simulink model "LabB_ObserverAndControllerOverRobot"  (R2023a)
settings: Solver=FixedStepDiscrete  StartTime=0.0  StopTime=inf  FixedStep=fSamplingPeriod  RelTol=1e-3  EnableMultiTasking=on
values from neighbouring files (symbols this model uses):
  Ad = [1 0 0 0 0.00216937580494 0.169257508882 0.0123862127288 3.63566071015 -3.56150302531e-05 -0.00954899425386 1.00059754622 0.218485145883 ... (16 elements, 4x4)]    [4_9.mat]    (also in IMPROVED_LQR_NUMRICAL.mat; LabB_ControllerOverSimulator_Discrete_Parameters.m = discreteStateSpace.A; LabB_ObserverAndControllerOverRobot_Parameters.m = [; LabB_ObserverAndControllerOverSimulator_Discrete_Parameters.m = discreteStateSpace.A)
  Bd = [0.000133880874091 0.0392918745799 -0.000585834385821 -0.17195692548]    [4_9.mat]    (also in IMPROVED_LQR_NUMRICAL.mat; LabB_ControllerOverSimulator_Discrete_Parameters.m = discreteStateSpace.B; LabB_ObserverAndControllerOverRobot_Parameters.m = [; LabB_ObserverAndControllerOverSimulator_Discrete_Parameters.m = discreteStateSpace.B)
  Cd = [1  0  0  0; 0  0  1  0]    [4_9.mat]    (also in IMPROVED_LQR_NUMRICAL.mat; LabB_ControllerOverSimulator_Discrete_Parameters.m = discreteStateSpace.C; LabB_ObserverAndControllerOverRobot_Parameters.m = [; LabB_ObserverAndControllerOverSimulator_Discrete_Parameters.m = discreteStateSpace.C)
  fGyroBias = -36.0405046481    [Copy_of_GyroBias.mat]    (also in GyroBias.mat; IMPROVED_LQR_NUMRICAL.mat = -55.293398533; PID_10_25.mat = -23.8864197531; PID_10_25_PROCESSED.mat = -23.8864197531)
  fGyroConversionFactor = 0.00762939453125    [IMPROVED_LQR_NUMRICAL.mat]    (also in LabB_ObserverAndControllerOverRobot_Parameters.m = -0.00763358778626; PID_10_25.mat = -0.00763358778626; PID_10_25_PROCESSED.mat = -0.00763358778626)
  fSamplingPeriod = 0.005    [4_10_numerical_derivative.mat]    (also in 4_9.mat; IMPROVED_LQR_NUMRICAL.mat; LabB_ControllerOverSimulator_Discrete_Parameters.m; LabB_ObserverAndControllerOverRobot_Parameters.m = 0.05)
  fWheelRadius = 0.0216    [IMPROVED_LQR_NUMRICAL.mat]    (also in LabB_ObserverAndControllerOverRobot_Parameters.m; PID_10_25.mat; PID_10_25_PROCESSED.mat)
  iNumberOfEncoderSteps = 720    [IMPROVED_LQR_NUMRICAL.mat]    (also in LabB_ObserverAndControllerOverRobot_Parameters.m; PID_10_25.mat; PID_10_25_PROCESSED.mat)
  Kd = -0.0902330229907    [4_8.mat]    (also in 4_8_LQR.mat; 4_9.mat = [-21.5910873349 -42.5517839322 -61.6884020442 -10.1567027547; IMPROVED_LQR_NUMRICAL.mat = [-21.5910873363 -42.5517839322 -61.6884020444 -10.1567027547; LabB_ControllerOverSimulator_Discrete_Parameters.m = acker(Ad,Bd,discretePoles))
  Ld = [0.113484873259  0.00523048580375; -1.36818722201  4.37324641743; 0.0236786814247  0.320119081479; 6.39094177477  -15.2655028264]    [4_9.mat]    (also in IMPROVED_LQR_NUMRICAL.mat = [0.14317878514  0.00902187336613; -0.912440934111  2.0839431; LabB_ObserverAndControllerOverRobot_Parameters.m = [; LabB_ObserverAndControllerOverSimulator_Discrete_Parameters.m = (place(Ad',Cd',desiredPoles))'; LabB_ObserverOverSimulator_Discrete_Parameters.m = (place(Ad',Cd',desiredPoles))')
  Md1 = [0.818659998491  0.0205458327288  0.00496425143631; 0.0212966370717  0.986017031865  0.0397631461808; -0.0224685177823  -0.180533078124  0.819806639231]    [4_9.mat]    (also in IMPROVED_LQR_NUMRICAL.mat = [0.852155353499  -0.0520013200777  0.00297877258471; -0.0532; LabB_ObserverAndControllerOverRobot_Parameters.m = [; LabB_ObserverAndControllerOverSimulator_Discrete_Parameters.m = Axx-Lacc*Ayx-Lnacc*Cx; LabB_ObserverOverSimulator_Discrete_Parameters.m = Axx-Lacc*Ayx-Lnacc*Cx)
  Md2 = [-8.22715382193e-05 0.0896973776791 -0.407469536485]    [4_9.mat]    (also in IMPROVED_LQR_NUMRICAL.mat = [-0.00455944705037 0.0553880900201 -0.371633068277]; LabB_ObserverAndControllerOverRobot_Parameters.m = [; LabB_ObserverAndControllerOverSimulator_Discrete_Parameters.m = Bx-Lacc*By; LabB_ObserverOverSimulator_Discrete_Parameters.m = Bx-Lacc*By)
  Md3 = [3.76127546986 376.495174844 -1759.12065562]    [4_9.mat]    (also in IMPROVED_LQR_NUMRICAL.mat = [-29.6802115428 120.227893263 -1491.44636344]; LabB_ObserverAndControllerOverRobot_Parameters.m = 1.0e+03 * [; LabB_ObserverAndControllerOverSimulator_Discrete_Parameters.m = Axy-Lacc*Ayy-Lnacc*Cy; LabB_ObserverOverSimulator_Discrete_Parameters.m = Axy-Lacc*Ayy-Lnacc*Cy)
  Md4 = [0.181803589786 -0.0442545183678 0.303604799034]    [4_9.mat]    (also in IMPROVED_LQR_NUMRICAL.mat = [0.14949925435 0.0394504885475 0.221851502925]; LabB_ObserverAndControllerOverRobot_Parameters.m = [; LabB_ObserverAndControllerOverSimulator_Discrete_Parameters.m = Lnacc; LabB_ObserverOverSimulator_Discrete_Parameters.m = Lnacc)
  Md5 = [-3.76127546986 -376.495174844 1759.12065562]    [4_9.mat]    (also in IMPROVED_LQR_NUMRICAL.mat = [29.6802115428 -120.227893263 1491.44636344]; LabB_ObserverAndControllerOverRobot_Parameters.m = 1.0e+03 * [; LabB_ObserverAndControllerOverSimulator_Discrete_Parameters.m = Lacc; LabB_ObserverOverSimulator_Discrete_Parameters.m = Lacc)
  Md6 = [1 0 0 0]    [4_9.mat]    (also in IMPROVED_LQR_NUMRICAL.mat; LabB_ObserverAndControllerOverRobot_Parameters.m = [; LabB_ObserverAndControllerOverSimulator_Discrete_Parameters.m = T(:,1); LabB_ObserverOverSimulator_Discrete_Parameters.m = T(:,1))
  Md7 = [0  0  0; 0  1  0; 1  0  0; 0  0  1]    [4_9.mat]    (also in IMPROVED_LQR_NUMRICAL.mat; LabB_ObserverAndControllerOverRobot_Parameters.m = [; LabB_ObserverAndControllerOverSimulator_Discrete_Parameters.m = T(:,2:4); LabB_ObserverOverSimulator_Discrete_Parameters.m = T(:,2:4))
undefined symbols (not defined in the file or in its folder): DiscIntNeverNeededParam
libraries: simulink x16, cstblocks x2, MinSegLibrary_M2V3 x2, arduinolib x1
settings Model: FPTRunName=FPA_Reference  SimulationMode=external  ExtModeTrigDuration=2  Creator=Alec  LastModifiedBy=Jasminis
settings SolverCC: AlgebraicLoopSolver=TrustRegion
settings DataIOCC: SaveFormat=Array  SaveOutput=off  SignalLogging=off  DSMLogging=off  SaveTime=off  ReturnWorkspaceOutputs=off
settings OptimizationCC: PassReuseOutputArgsAs=Individual arguments  ExpressionDepthLimit=2147483647  MaxStackSize=64  EfficientTunableParamExpr=on
settings DebuggingCC: UnderspecifiedInitializationDetection=Classic  MergeDetectMultiDrivingBlocksExec=none  ParameterTunabilityLossMsg=error  UnconnectedInputMsg=warning  UnconnectedOutputMsg=warning  UnconnectedLineMsg=warning  StateNameClashWarn=warning  SFUnexpectedBacktrackingDiag=warning  SFNoUnconditionalDefaultTransitionDiag=warning  SFExecutionAtInitializationDiag=none  ArithmeticOperatorsInVariantConditions=warning
settings HardwareCC: ProdBitPerInt=16  ProdBitPerPointer=16  ProdBitPerSizeT=16  ProdBitPerPtrDiffT=16  ProdLargestAtomicFloat=None  ProdWordSize=8  ProdHWDeviceType=Atmel->AVR
settings ModelReferenceCC: EnableRefExpFcnMdlSchedulingChecks=on  PropagateSignalLabelsOutOfModel=off
settings SFSimCC: SimUseLocalCustomCode=off  MATLABDynamicMemAlloc=off  CustomCodeUndefinedFunction=UseInterfaceOnly
settings RTWCC: Description=Embedded Coder  SystemTargetFile=ert.tlc  HardwareBoard=Arduino Mega 2560  TemplateMakefile=ert_default_tmf  GenerateReport=on  RTWVerbose=off  RTWUseLocalCustomCode=off  Toolchain=Arduino AVR  BuildConfiguration=Faster Runs  IncludeHyperlinkInReport=on  LaunchReport=on  GenerateTraceInfo=on  GenerateTraceReport=on  GenerateTraceReportSl=on  GenerateTraceReportSf=on  GenerateTraceReportEml=on
settings CodeAppCC: ForceParamTrailComments=on  IgnoreCustomStorageClasses=off  OperatorAnnotations=on  SimulinkDataObjDesc=on  SFDataObjDesc=on  MATLABFcnDesc=on  CustomSymbolStrType=$N$R$M  InsertBlockDesc=on  StateflowObjectComments=on  MATLABSourceComments=on  InternalIdentifier=Classic
settings ERTTargetCC: SupportContinuousTime=on  SupportVariableSizeSignals=on
settings ConfigComp: CovMetricSettings=dw  CovSaveCumulativeToWorkspaceVar=on  CovSaveSingleToWorkspaceVar=on  CovExternalEMLEnable=off

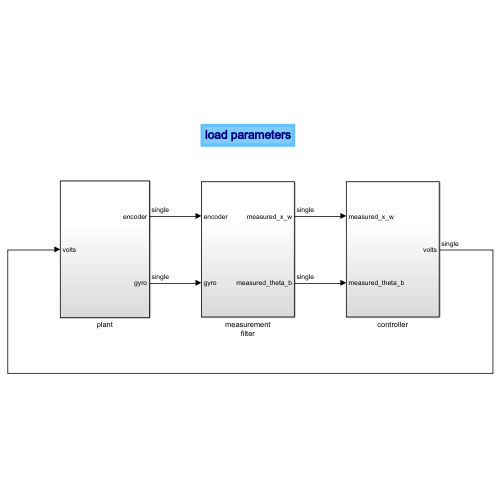
[thumbnail: Simulink's stored preview of the top-level diagram]
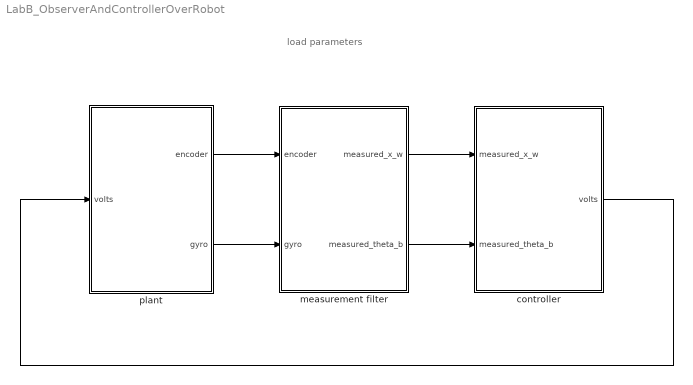
== system LabB_ObserverAndControllerOverRobot ==
  note: load parameters
  controller : Subsystem
  measurement filter : Subsystem
  plant : Subsystem
  wires:
  plant/2(gyro) -> measurement filter/2(gyro)
  measurement filter/2(measured_theta_b) -> controller/2("measured_theta_b ")
  measurement filter/1(measured_x_w) -> controller/1(measured_x_w)
  plant/1(encoder) -> measurement filter/1(encoder)
  controller/1(volts) -> plant/1(volts)

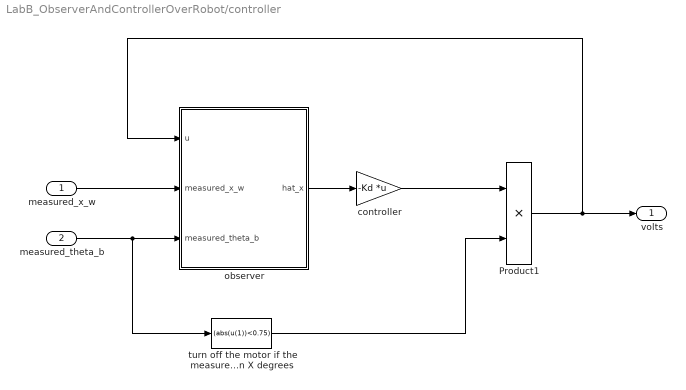
== system LabB_ObserverAndControllerOverRobot/controller ==
  measured_x_w : Inport
  "measured_theta_b " : Inport  Port=2
  Product1 : Product  RndMeth=Zero
  controller : Gain  Gain=-Kd  Multiplication=Matrix(K*u)
  observer : Subsystem
  turn off the motor if the measured angle is greater than X degrees : Fcn  Expr=(abs(u(1))<0.75)
  volts : Outport
  wires:
  observer/1(hat_x) -> controller/1
  turn off the motor if the measured angle is greater than X degrees/1 -> Product1/2
  "measured_theta_b "/1 -> observer/3(measured_theta_b), turn off the motor if the measured angle is greater than X degrees/1
  controller/1 -> Product1/1
  measured_x_w/1 -> observer/2(measured_x_w)
  Product1/1 -> observer/1(u), volts/1

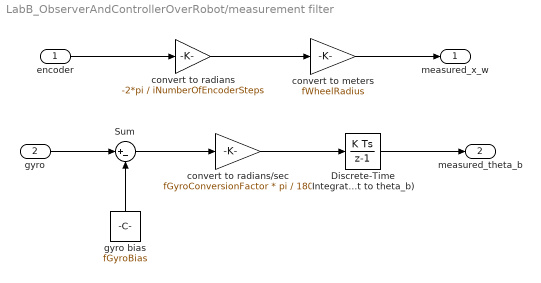
== system LabB_ObserverAndControllerOverRobot/measurement filter ==
  encoder : Inport
  gyro : Inport  Port=2
  Discrete-Time Integrator (convert from theta_b_dot to theta_b) : DiscreteIntegrator  SampleTime=fSamplingPeriod  OutDataTypeStr=Inherit: Inherit via back propagation  ICPrevOutput=DiscIntNeverNeededParam  ICPrevScaledInput=DiscIntNeverNeededParam
  Sum : Sum  Inputs=|+-
  convert to radians/sec : Gain  Gain=fGyroConversionFactor * pi / 180  OutDataTypeStr=Inherit: Same as input
  convert to radians : Gain  Gain=-2*pi / iNumberOfEncoderSteps  OutDataTypeStr=Inherit: Same as input
  convert to meters : Gain  Gain=fWheelRadius  OutDataTypeStr=Inherit: Same as input
  gyro bias : Constant  Value=fGyroBias  OutDataTypeStr=single
  measured_x_w : Outport
  measured_theta_b : Outport  Port=2
  wires:
  convert to radians/sec/1 -> Discrete-Time Integrator (convert from theta_b_dot to theta_b)/1
  gyro/1 -> Sum/1
  Sum/1 -> convert to radians/sec/1
  convert to radians/1 -> convert to meters/1
  encoder/1 -> convert to radians/1
  Discrete-Time Integrator (convert from theta_b_dot to theta_b)/1 -> measured_theta_b/1
  gyro bias/1 -> Sum/2
  convert to meters/1 -> measured_x_w/1

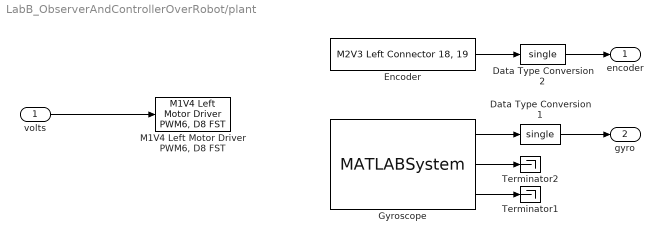
== system LabB_ObserverAndControllerOverRobot/plant ==
  volts : Inport
  Data Type Conversion1 : DataTypeConversion  OutDataTypeStr=single  SaturateOnIntegerOverflow=off  RndMeth=Floor
  Data Type Conversion2 : DataTypeConversion  OutDataTypeStr=single  SaturateOnIntegerOverflow=off  RndMeth=Floor
  Encoder : MinSegLibrary_M2V3/M2V3 Left Connector 18, 19  Encoder=1  PinA=19  PinB=18
      settings: SourceProductName=Rensselaer Arduino Support Package
  Gyroscope : MATLABSystem  System=soMPU6050Gyro  DLPFmode=0
      mask Type: soMPU6050Gyro
      mask Display:
      | disp('soMPU6050Gyro');
      | port_label('output',1,'xvel');
      | port_label('output',2,'yvel');
      | port_label('output',3,'zvel');
  "M1V4 Left Motor Driver PWM6, D8 FST" : MinSegLibrary_M2V3/M1V4 Left Motor Driver PWM6, D8 FST  Vsupply=9
      settings: SourceProductName=Rensselaer Arduino Support Package
  Terminator1 : Terminator
  Terminator2 : Terminator
  encoder : Outport
  gyro : Outport  Port=2
  wires:
  Gyroscope/1 -> Data Type Conversion1/1
  Data Type Conversion1/1 -> gyro/1
  Encoder/1 -> Data Type Conversion2/1
  Data Type Conversion2/1 -> encoder/1
  Gyroscope/3 -> Terminator1/1
  Gyroscope/2 -> Terminator2/1
  volts/1 -> "M1V4 Left Motor Driver PWM6, D8 FST"/1

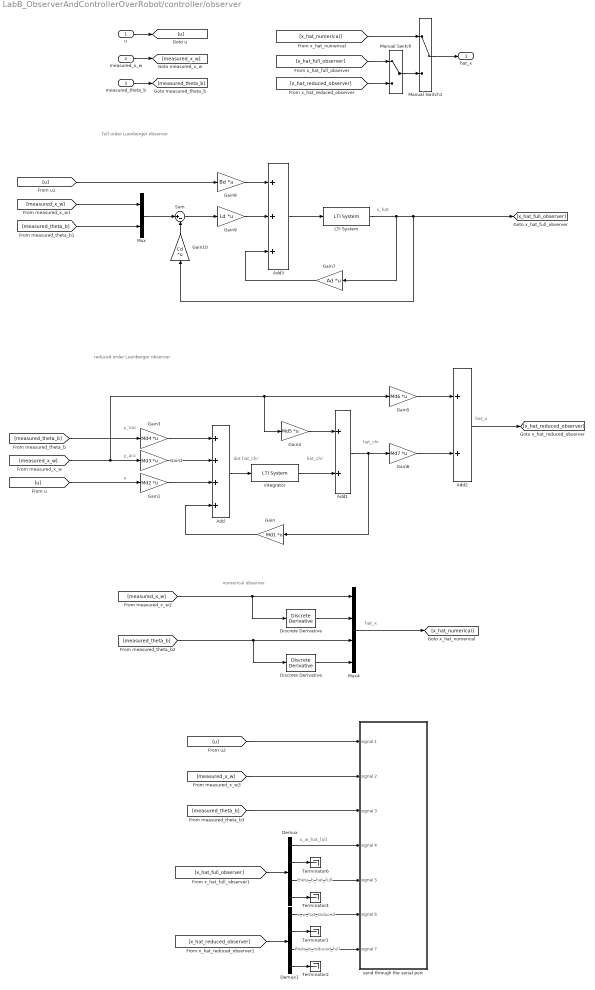
== system LabB_ObserverAndControllerOverRobot/controller/observer ==
  note: x_w_hat_full
  note: full order Luenberger observer
  note: reduced order Luenberger observer
  note: numerical observer
  note: hat_x
  note: hat_chi
  note: u
  note: dot hat_chi'
  note: hat_chi'
  note: y_acc
  note: y_nac
  note: x_hat
  note: hat_x
  note: x_w_hat_reduced
  note: theta_b_hat_full
  note: theta_b_reduced_full
  u : Inport
  measured_x_w : Inport  Port=2
  measured_theta_b : Inport  Port=3
  Add : Sum  Inputs=++++
  Add1 : Sum
  Add2 : Sum
  Add3 : Sum  Inputs=+++
  Demux : Demux
  Demux1 : Demux
  Discrete Derivative : simulink/Discrete/Discrete Derivative  gainval=1.0  ICPrevScaledInput=0.0  OutMin=[]  OutMax=[]  OutDataType=fixdt(1, 16)  OutScaling=2^-10  DoSatur=off
  "Discrete Derivative " : simulink/Discrete/Discrete Derivative  gainval=1.0  ICPrevScaledInput=0.0  OutMin=[]  OutMax=[]  OutDataType=fixdt(1, 16)  OutScaling=2^-10  DoSatur=off
  Gain : Gain  Gain=Md1  Multiplication=Matrix(K*u)
  Gain1 : Gain  Gain=Md2  Multiplication=Matrix(K*u)
  Gain10 : Gain  Gain=Cd  Multiplication=Matrix(K*u)
  Gain2 : Gain  Gain=Md3  Multiplication=Matrix(K*u)
  Gain3 : Gain  Gain=Md4  Multiplication=Matrix(K*u)
  Gain4 : Gain  Gain=Md5  Multiplication=Matrix(K*u)
  Gain5 : Gain  Gain=Md6  Multiplication=Matrix(K*u)
  Gain6 : Gain  Gain=Md7  Multiplication=Matrix(K*u)
  Gain7 : Gain  Gain=Ad  Multiplication=Matrix(K*u)
  Gain8 : Gain  Gain=Bd  Multiplication=Matrix(K*u)
  Gain9 : Gain  Gain=Ld  Multiplication=Matrix(K*u)
  LTI System : cstblocks/LTI System  sys=tf(1,[1 0],fSamplingPeriod)*eye(size(Ad))  IC=[]
  Manual Switch : ManualSwitch
  Manual Switch1 : ManualSwitch
  Mux : Mux  Inputs=2
  Mux4 : Mux
  Sum : Sum  Inputs=|+-
  Terminator{1..2,4,6} (4 alike) : Terminator
  integrator : cstblocks/LTI System  sys=tf(1,[1 0],fSamplingPeriod)*eye(3)  IC=[]
  send through the serial port : Subsystem
  hat_x : Outport
  wires:
  Gain3/1 -> Add/1
  Gain2/1 -> Add/2
  Add/1 -> integrator/1
  Gain4/1 -> Add1/1
  Gain1/1 -> Add/3
  Gain/1 -> Add/4
  integrator/1 -> Add1/2
  Add1/1 -> Gain/1, Gain6/1
  Gain5/1 -> Add2/1
  Gain6/1 -> Add2/2
  Discrete Derivative/1 -> Mux4/2
  "Discrete Derivative "/1 -> Mux4/4
  [measured_x_w] -> Gain4/1, Gain5/1, Gain2/1
  [measured_theta_b] -> Gain3/1
  Gain9/1 -> Add3/2
  Sum/1 -> Gain9/1
  [u] -> Gain1/1
  Gain8/1 -> Add3/1
  Gain10/1 -> Sum/2
  Mux/1 -> Sum/1
  Gain7/1 -> Add3/3
  LTI System/1 -> [x_hat_full_observer], Gain10/1, Gain7/1
  Add3/1 -> LTI System/1
  u/1 -> [u]
  measured_x_w/1 -> [measured_x_w]
  measured_theta_b/1 -> [measured_theta_b]
  [u] -> Gain8/1
  [measured_x_w] -> Mux/1
  [measured_theta_b] -> Mux/2
  [measured_x_w] -> Discrete Derivative/1, Mux4/1
  [measured_theta_b] -> "Discrete Derivative "/1, Mux4/3
  [u] -> send through the serial port/1(signal 1)
  [measured_x_w] -> send through the serial port/2(signal 2)
  [measured_theta_b] -> send through the serial port/3(signal 3)
  Mux4/1 -> [x_hat_numerical]
  [x_hat_full_observer] -> Manual Switch/1
  Manual Switch/1 -> Manual Switch1/2
  Manual Switch1/1 -> hat_x/1
  Add2/1 -> [x_hat_reduced_observer]
  [x_hat_reduced_observer] -> Manual Switch/2
  [x_hat_numerical] -> Manual Switch1/1
  [x_hat_full_observer] -> Demux/1
  Demux/1 -> send through the serial port/4(signal 4)
  Demux/3 -> send through the serial port/5(signal 5)
  Demux1/3 -> send through the serial port/7(signal 7)
  Demux1/1 -> send through the serial port/6(signal 6)
  [x_hat_reduced_observer] -> Demux1/1
  Demux/2 -> Terminator6/1
  Demux/4 -> Terminator4/1
  Demux1/2 -> Terminator1/1
  Demux1/4 -> Terminator2/1

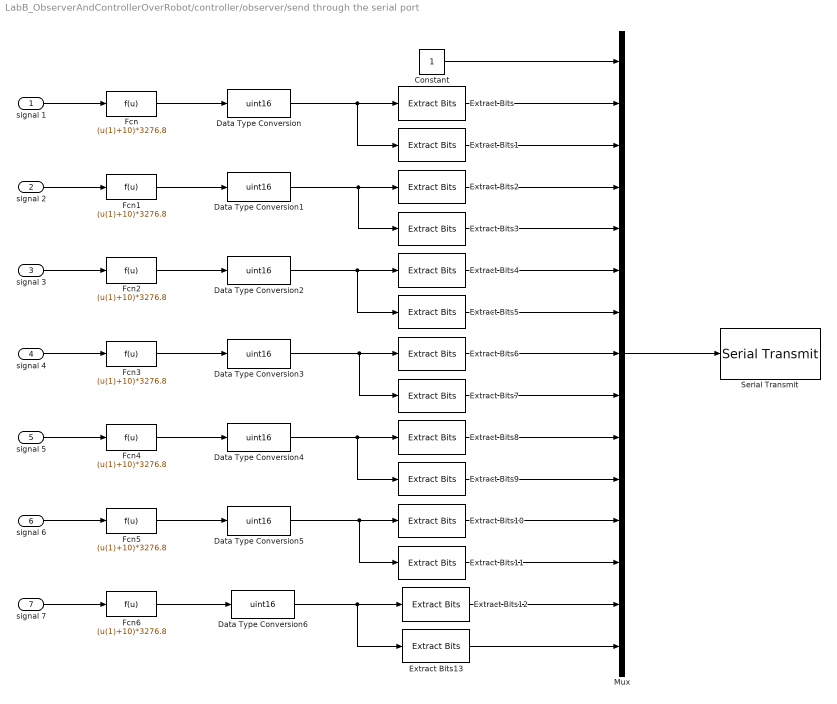
== system LabB_ObserverAndControllerOverRobot/controller/observer/send through the serial port ==
  signal 1 : Inport
  signal 2 : Inport  Port=2
  signal 3 : Inport  Port=3
  signal 4 : Inport  Port=4
  signal 5 : Inport  Port=5
  signal 6 : Inport  Port=6
  signal 7 : Inport  Port=7
  Constant : Constant  OutDataTypeStr=uint8
  Data Type Conversion{,1..6} (7 alike) : DataTypeConversion  OutDataTypeStr=uint16  SaturateOnIntegerOverflow=off  RndMeth=Floor
  Extract Bits{,2,4,6,8,10,12} (7 alike) : simulink/Logic and Bit Operations/Extract Bits  bitsToExtract=Upper half  numBits=8  bitIdxRange=[0 7]  outScalingMode=Treat bit field as an integer
  Extract Bits{1,3,5,7,9,11,13} (7 alike) : simulink/Logic and Bit Operations/Extract Bits  bitsToExtract=Lower half  numBits=8  bitIdxRange=[0 7]  outScalingMode=Treat bit field as an integer
  Fcn{,1..6} (7 alike) : Fcn  Expr=(u(1)+10)*3276.8
  Mux : Mux  Inputs=15
  Serial Transmit : arduinolib/Serial Transmit  portNumber=0  sendmode=write  sendformat=Decimal  floatprecision=2  blockPlatform=arduino
  wires:
  Data Type Conversion/1 -> Extract Bits1/1, Extract Bits/1
  Extract Bits/1 -> Mux/2
  Fcn1/1 -> Data Type Conversion1/1
  Fcn/1 -> Data Type Conversion/1
  Extract Bits2/1 -> Mux/4
  Constant/1 -> Mux/1
  Data Type Conversion1/1 -> Extract Bits2/1, Extract Bits3/1
  Extract Bits1/1 -> Mux/3
  Mux/1 -> Serial Transmit/1
  Extract Bits3/1 -> Mux/5
  Data Type Conversion3/1 -> Extract Bits6/1, Extract Bits7/1
  Extract Bits4/1 -> Mux/6
  Data Type Conversion2/1 -> Extract Bits5/1, Extract Bits4/1
  Extract Bits5/1 -> Mux/7
  Extract Bits6/1 -> Mux/8
  Fcn3/1 -> Data Type Conversion3/1
  Extract Bits7/1 -> Mux/9
  Fcn2/1 -> Data Type Conversion2/1
  Data Type Conversion4/1 -> Extract Bits9/1, Extract Bits8/1
  Fcn5/1 -> Data Type Conversion5/1
  Extract Bits8/1 -> Mux/10
  Extract Bits9/1 -> Mux/11
  Data Type Conversion5/1 -> Extract Bits10/1, Extract Bits11/1
  Extract Bits11/1 -> Mux/13
  Extract Bits10/1 -> Mux/12
  Fcn4/1 -> Data Type Conversion4/1
  signal 2/1 -> Fcn1/1
  signal 7/1 -> Fcn6/1
  signal 6/1 -> Fcn5/1
  signal 3/1 -> Fcn2/1
  signal 1/1 -> Fcn/1
  signal 4/1 -> Fcn3/1
  signal 5/1 -> Fcn4/1
  Extract Bits13/1 -> Mux/15
  Extract Bits12/1 -> Mux/14
  Fcn6/1 -> Data Type Conversion6/1
  Data Type Conversion6/1 -> Extract Bits12/1, Extract Bits13/1
